simulink model "DR_DigitalTwin"  (R2026a)
settings: Solver=VariableStepAuto  StopTime=1000
undefined symbols (not defined in the file): m
settings Model: Creator=dell  LastModifiedBy=dell

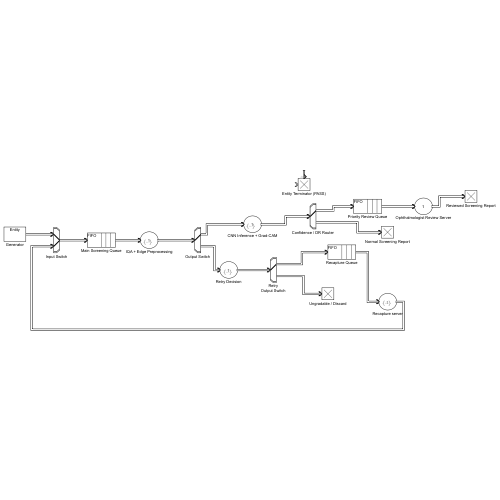
[thumbnail: Simulink's stored preview of the top-level diagram]
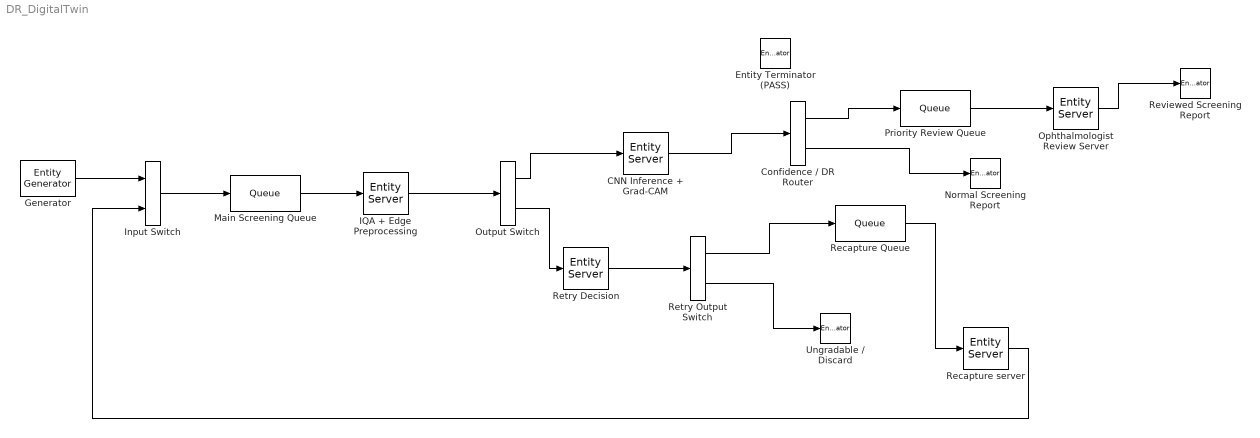
== system DR_DigitalTwin ==
  CNN Inference + Grad-CAM : EntityServer  InputPortMessageModes=m  OutputPortMessageModes=m  Capacity=1  ServiceTimeValue=ai_processing_time  ServiceCompleteAction=|
      | % Decide whether human review is needed
      | if entity.confidence_level == 3 || entity.dr_severity >= 2
      |     entity.review_route = 2;
      | else
      |     entity.review_route = 1;
      | end
      | 
      | % Assign review priority
      | if entity.dr_severity >= 3
      |     entity.review_priority = 3;
      | elseif entity.dr_severity >= 2 || entity.confidence_level == 3
      |     entity.review_priority = 2;
      | else
      |     entity.review_priority = 1;
      | end
  Confidence / DR Router : EntityOutputSwitch  InputPortMessageModes=m  OutputPortMessageModes=m,m  SwitchingCriterion=From attribute  SwitchAttributeName=retry_route
  Entity Terminator (PASS) : EntityTerminator  InputPortMessageModes=m  NumberEntitiesArrived=on
      settings: OutputPortMap=o0
  Generator : EntityGenerator  OutputPortMessageModes=m  TimeSource=MATLAB action  IntergenerationTimeAction=dt = -(1/arrival_rate)*log(1-rand());  AttributeName=retry_count|iqa_status|dr_severity|confidence_level|iqa_route|retry_route|review_route|review_priority  AttributeInitialValue=0|test_iqa_status|test_dr_severity|test_confidence_level|1|1|1|1  EntityType=Structured  EntityTypeName=Entity
  IQA + Edge Preprocessing : EntityServer  InputPortMessageModes=m  OutputPortMessageModes=m  Capacity=1  ServiceTimeValue=2  ServiceCompleteAction=entity.iqa_route = entity.iqa_status + 1;
  Input Switch : EntityInputSwitch  InputPortMessageModes=m,m  OutputPortMessageModes=m
  Main Screening Queue : Queue  InputPortMessageModes=m  OutputPortMessageModes=m
  Normal Screening Report : EntityTerminator  InputPortMessageModes=m
  Ophthalmologist Review Server : EntityServer  InputPortMessageModes=m  OutputPortMessageModes=m  Capacity=1  ServiceTimeValue=review_processing_time
  Output Switch : EntityOutputSwitch  InputPortMessageModes=m  OutputPortMessageModes=m,m  SwitchingCriterion=From attribute  SwitchAttributeName=iqa_route
  Priority Review Queue : Queue  InputPortMessageModes=m  OutputPortMessageModes=m
  Recapture Queue : Queue  InputPortMessageModes=m  OutputPortMessageModes=m
  Recapture server : EntityServer  InputPortMessageModes=m  OutputPortMessageModes=m  Capacity=1  ServiceCompleteAction=entity.retry_count = entity.retry_count + 1;
  Retry Output Switch : EntityOutputSwitch  InputPortMessageModes=m  OutputPortMessageModes=m,m  SwitchingCriterion=From attribute  SwitchAttributeName=retry_route
  Retry Decision : EntityServer  InputPortMessageModes=m  OutputPortMessageModes=m  Capacity=1  ServiceCompleteAction=|
      | if entity.retry_count < max_retries
      |     entity.retry_route = 1;
      | else
      |     entity.retry_route = 2;
      | end
  Reviewed Screening Report : EntityTerminator  InputPortMessageModes=m
  Ungradable / Discard : EntityTerminator  InputPortMessageModes=m
  wires:
  Input Switch/1 -> Main Screening Queue/1
  Output Switch/1 -> CNN Inference + Grad-CAM/1
  Recapture Queue/1 -> Recapture server/1
  Generator/1 -> Input Switch/1
  Output Switch/2 -> Retry Decision/1
  Recapture server/1 -> Input Switch/2
  Main Screening Queue/1 -> IQA + Edge Preprocessing/1
  IQA + Edge Preprocessing/1 -> Output Switch/1
  Retry Decision/1 -> Retry Output Switch/1
  Retry Output Switch/1 -> Recapture Queue/1
  Retry Output Switch/2 -> Ungradable / Discard/1
  CNN Inference + Grad-CAM/1 -> Confidence / DR Router/1
  Confidence / DR Router/1 -> Priority Review Queue/1
  Priority Review Queue/1 -> Ophthalmologist Review Server/1
  Confidence / DR Router/2 -> Normal Screening Report/1
  Ophthalmologist Review Server/1 -> Reviewed Screening Report/1
